simulink model "simul_observ"  (R2021b)
settings: Solver=VariableStepAuto  StartTime=0.0  StopTime=10.0  RelTol=1e-3
values from neighbouring files (symbols this model uses):
  A = [0 1 0 0 ... (first row only)    [q13.m]    (also in q21.m)
  B = [0; 0; 0; 1/J]    [q13.m]    (also in q21.m)
  C = [1 0 0 0 ... (first row only)    [q13.m]    (also in q21.m)
  K = place(A,B,P)    [q13.m]    (also in q21.m = lqr(A,B,R,Q); q8.m = [0 0 0 0])
  L = place(A',C',PL)'    [q21.m]
settings Model: Creator=Arthur  LastModifiedBy=Arthur
settings DataIOCC: ExternalInput=Rref  SaveFormat=Array

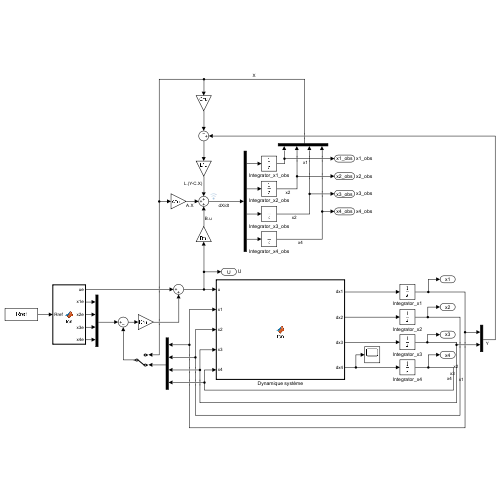
[thumbnail: Simulink's stored preview of the top-level diagram]
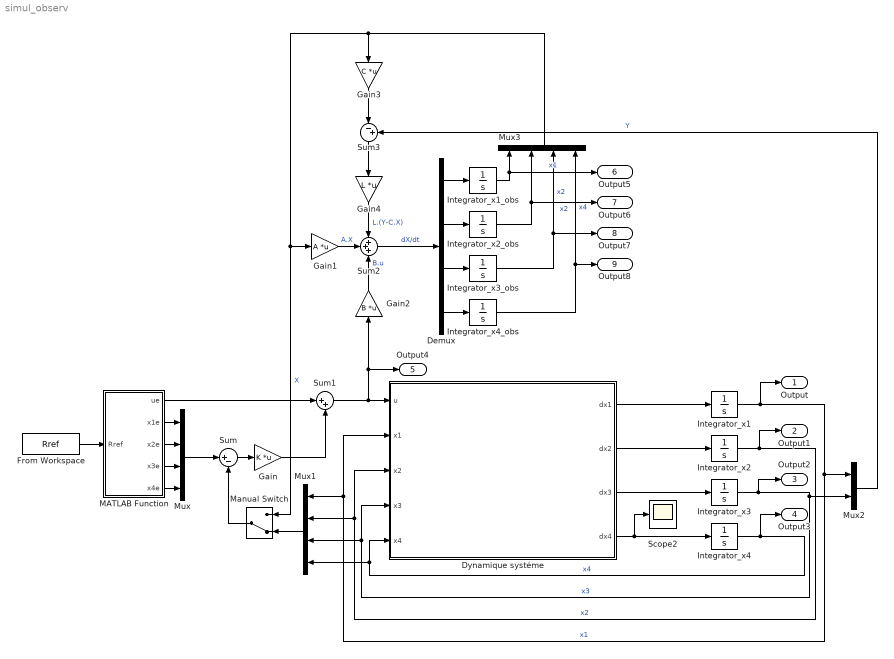
== system simul_observ ==
  Demux : Demux
  Dynamique systéme : MATLAB Function  TreatAsAtomicUnit=on
  From Workspace : FromWorkspace  VariableName=Rref  OutDataTypeStr=double  SampleTime=0.01
  Gain : Gain  Gain=K  Multiplication=Matrix(K*u)
  Gain1 : Gain  Gain=A  Multiplication=Matrix(K*u)
  Gain2 : Gain  Gain=B  Multiplication=Matrix(K*u)
  Gain3 : Gain  Gain=C  Multiplication=Matrix(K*u)
  Gain4 : Gain  Gain=L  Multiplication=Matrix(K*u)
  Integrator_x1 : Integrator  InitialCondition=0.1
  Integrator_x1_obs : Integrator
  Integrator_x2 : Integrator
  Integrator_x2_obs : Integrator
  Integrator_x3 : Integrator
  Integrator_x3_obs : Integrator
  Integrator_x4 : Integrator
  Integrator_x4_obs : Integrator
  MATLAB Function : MATLAB Function  TreatAsAtomicUnit=on
  Manual Switch : ManualSwitch  CurrentSetting=0
  Mux : Mux
  Mux1 : Mux
  Mux2 : Mux  Inputs=2
  Mux3 : Mux
  Scope2 : Scope
  Sum : Sum  Inputs=|+-
  Sum1 : Sum  Inputs=|++
  Sum2 : Sum  Inputs=+++
  Sum3 : Sum  Inputs=|-+
  Output : Outport
  Output1 : Outport  Port=2
  Output2 : Outport  Port=3
  Output3 : Outport  Port=4
  Output4 : Outport  Port=5  SignalName=U
  Output5 : Outport  Port=6  SignalName=x1_obs
  Output6 : Outport  Port=7  SignalName=x2_obs
  Output7 : Outport  Port=8  SignalName=x3_obs
  Output8 : Outport  Port=9  SignalName=x4_obs
  wires:
  Dynamique systéme/1(dx1) -> Integrator_x1/1
  Dynamique systéme/2(dx2) -> Integrator_x2/1
  Dynamique systéme/3(dx3) -> Integrator_x3/1
  Dynamique systéme/4(dx4) -> Scope2/1, Integrator_x4/1
  Integrator_x4/1 -> Output3/1, Mux1/4, Dynamique systéme/5(x4)  "x4"
  Integrator_x3/1 -> Mux1/3, Dynamique systéme/4(x3), Mux2/2, Output2/1  "x3"
  Integrator_x2/1 -> Mux1/2, Dynamique systéme/3(x2), Output1/1  "x2"
  Integrator_x1/1 -> Mux1/1, Dynamique systéme/2(x1), Mux2/1, Output/1  "x1"
  MATLAB Function/2(x1e) -> Mux/1
  MATLAB Function/3(x2e) -> Mux/2
  MATLAB Function/4(x3e) -> Mux/3
  MATLAB Function/5(x4e) -> Mux/4
  Mux/1 -> Sum/1
  Sum/1 -> Gain/1
  Sum1/1 -> Dynamique systéme/1(u), Gain2/1, Output4/1
  MATLAB Function/1(ue) -> Sum1/1
  From Workspace/1 -> MATLAB Function/1(Rref)
  Gain/1 -> Sum1/2
  Gain1/1 -> Sum2/2  "A.X"
  Gain2/1 -> Sum2/3  "B.u"
  Gain4/1 -> Sum2/1  "L.(Y-C.X)"
  Sum3/1 -> Gain4/1
  Sum2/1 -> Demux/1  "dX/dt"
  Demux/1 -> Integrator_x1_obs/1
  Demux/2 -> Integrator_x2_obs/1
  Demux/3 -> Integrator_x3_obs/1
  Demux/4 -> Integrator_x4_obs/1
  Integrator_x4_obs/1 -> Mux3/4, Output8/1  "x4"
  Integrator_x3_obs/1 -> Mux3/3, Output7/1  "x2"
  Integrator_x2_obs/1 -> Mux3/2, Output6/1  "x2"
  Integrator_x1_obs/1 -> Mux3/1, Output5/1  "x1"
  Mux3/1 -> Gain3/1, Manual Switch/1, Gain1/1  "X"
  Mux2/1 -> Sum3/2  "Y"
  Gain3/1 -> Sum3/1
  Manual Switch/1 -> Sum/2
  Mux1/1 -> Manual Switch/2

== matlab function simul_observ/MATLAB Function ==
  data: Rref input; ue output; x1e output; x2e output; x3e output; x4e output
function [ue,x1e,x2e,x3e,x4e] = fcn(Rref)
    % declaration constants
    m = 0.6; % kg
    g = 9.81; % m/s^2

    x1e = Rref;
    x2e = 0;
    x3e = 0;
    x4e = 0;
    ue = m*g*x1e;

== matlab function simul_observ/Dynamique systéme ==
  data: u input; dx1 output; x1 input; x2 input; x3 input; x4 input; dx2 output; dx3 output; dx4 output
function [dx1,dx2,dx3,dx4] = fcn(u,x1,x2,x3,x4)
    % declaration constants
    J = 0.02; % kg.m^2
    m = 0.6; % kg
    sigma = 0.8; % adimentional
    g = 9.81; % m/s^2
    
    % dynamique
    dx1 = x2;
    dx2 = (x1*x4*x4-g*sin(x3))/(1+sigma);
    dx3 = x4;
    dx4 = (u-m*g*x1*cos(x3)-2*m*x1*x2*x4)/(J+m*x1*x1);
